simulink model "a"  (R2018b)
settings: Solver=VariableStepAuto  StartTime=0.0  StopTime=30  RelTol=1e-6
values from neighbouring files (symbols this model uses):
  H0 = 1000    [init.m]
  m = 100    [init.m]
  V0 = 250    [init.m]
undefined symbols (not defined in the file or in its folder): alfa, G, p, Wx, Wz, x0, Y, z0
libraries: simulink x1
settings Model: Creator=cool  LastModifiedBy=cool

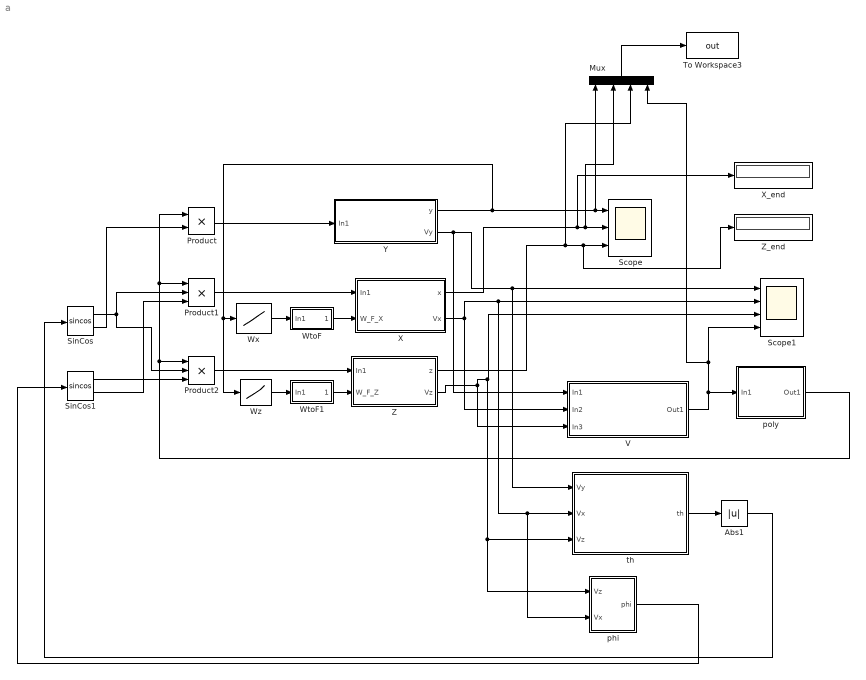
== system a ==
  Abs1 : Abs
  Mux : Mux
  Product : Product
  Product1 : Product  Inputs=3
  Product2 : Product  Inputs=3
  Scope : Scope  NumInputPorts=3
  Scope1 : Scope  NumInputPorts=4
  SinCos : Trigonometry  Operator=sincos
  SinCos1 : Trigonometry  Operator=sincos
  To Workspace3 : ToWorkspace  VariableName=out  SaveFormat=Timeseries  SampleTime=-1
  V : Subsystem
  WtoF : Subsystem
  WtoF1 : Subsystem
  Wx : Lookup_n-D  NumberOfTableDimensions=1  BreakpointsForDimension1=Y  Table=Wx  InterpMethod=Cubic spline  InternalRulePriority=Speed  RndMeth=Simplest  InputSameDT=on
  Wz : Lookup_n-D  NumberOfTableDimensions=1  BreakpointsForDimension1=Y  Table=Wz  InterpMethod=Cubic spline  InternalRulePriority=Speed  RndMeth=Simplest  InputSameDT=on
  X : Subsystem
  X_end : Display
  Y : Subsystem
  Z : Subsystem
  Z_end : Display
  "phi " : Subsystem
  "poly " : Subsystem
  th : Subsystem
  wires:
  Y/1(y) -> Wx/1, Wz/1, Scope/1, Mux/1
  X/1(x) -> Mux/2, Scope/2, X_end/1
  Z/1(z) -> Mux/3, Z_end/1, Scope/3
  Y/2(Vy) -> V/1(In1), th/1(Vy), Scope1/1
  X/2(Vx) -> "phi "/2(Vx), th/2(Vx), Scope1/2, V/2(In2)
  Z/2(Vz) -> "phi "/1(Vz), th/3(Vz), Scope1/3, V/3(In3)
  V/1(Out1) -> "poly "/1(In1), Mux/4, Scope1/4
  "poly "/1(Out1) -> Product2/1, Product/1, Product1/1
  th/1(th) -> Abs1/1
  SinCos/2 -> Product/2
  SinCos/1 -> Product1/2, Product2/2
  Product/1 -> Y/1(In1)
  Product2/1 -> Z/1(In1)
  Product1/1 -> X/1(In1)
  "phi "/1(phi) -> SinCos1/1
  Abs1/1 -> SinCos/1
  SinCos1/2 -> Product1/3
  SinCos1/1 -> Product2/3
  Mux/1 -> To Workspace3/1
  Wx/1 -> WtoF/1(In1)
  WtoF/1(Out1) -> X/2(W_F_X)
  Wz/1 -> WtoF1/1(In1)
  WtoF1/1(Out1) -> Z/2(W_F_Z)

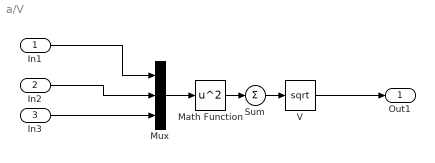
== system a/V ==
  In1 : Inport
  In2 : Inport  Port=2
  In3 : Inport  Port=3
  Math Function : Math  Operator=square  SaturateOnIntegerOverflow=on
  Mux : Mux  Inputs=3
  Sum : Sum  Inputs=+
  V : Sqrt  SaturateOnIntegerOverflow=on
  Out1 : Outport
  wires:
  Mux/1 -> Math Function/1
  In3/1 -> Mux/3
  Math Function/1 -> Sum/1
  In2/1 -> Mux/2
  Sum/1 -> V/1
  In1/1 -> Mux/1
  V/1 -> Out1/1

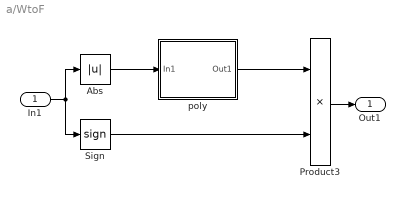
== system a/WtoF ==
  In1 : Inport
  Abs : Abs
  Product3 : Product
  Sign : Signum
  "poly " : Subsystem
  Out1 : Outport
  wires:
  In1/1 -> Sign/1, Abs/1
  Product3/1 -> Out1/1
  Sign/1 -> Product3/2
  Abs/1 -> "poly "/1(In1)
  "poly "/1(Out1) -> Product3/1

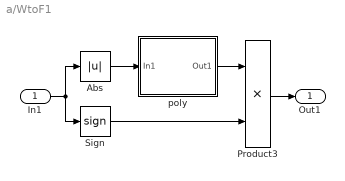
== system a/WtoF1 ==
  In1 : Inport
  Abs : Abs
  Product3 : Product
  Sign : Signum
  "poly " : Subsystem
  Out1 : Outport
  wires:
  Sign/1 -> Product3/2
  Product3/1 -> Out1/1
  In1/1 -> Abs/1, Sign/1
  "poly "/1(Out1) -> Product3/1
  Abs/1 -> "poly "/1(In1)

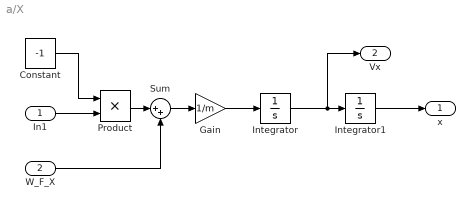
== system a/X ==
  In1 : Inport
  W_F_X : Inport  Port=2
  Constant : Constant  Value=-1
  Gain : Gain  Gain=1/m
  Integrator : Integrator  InitialCondition=V0*cos(alfa)
  Integrator1 : Integrator  InitialCondition=x0
  Product : Product
  Sum : Sum  Inputs=|++
  x : Outport
  Vx : Outport  Port=2
  wires:
  Integrator1/1 -> x/1
  Gain/1 -> Integrator/1
  In1/1 -> Product/2
  Constant/1 -> Product/1
  Integrator/1 -> Vx/1, Integrator1/1
  Product/1 -> Sum/1
  Sum/1 -> Gain/1
  W_F_X/1 -> Sum/2

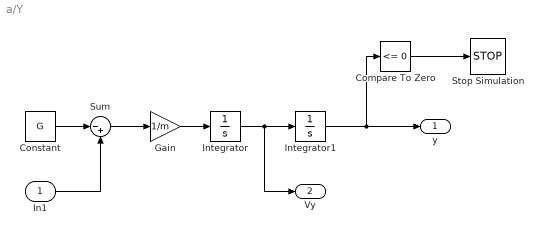
== system a/Y ==
  In1 : Inport
  Compare To Zero : simulink/Logic and Bit Operations/Compare To Zero  relop=<=  OutDataTypeStr=boolean
  Constant : Constant  Value=G
  Gain : Gain  Gain=1/m
  Integrator : Integrator
  Integrator1 : Integrator  InitialCondition=H0
  Stop Simulation : Stop
  Sum : Sum  Inputs=|-+
  y : Outport
  Vy : Outport  Port=2
  wires:
  Gain/1 -> Integrator/1
  Compare To Zero/1 -> Stop Simulation/1
  Integrator1/1 -> Compare To Zero/1, y/1
  Sum/1 -> Gain/1
  Constant/1 -> Sum/1
  In1/1 -> Sum/2
  Integrator/1 -> Vy/1, Integrator1/1

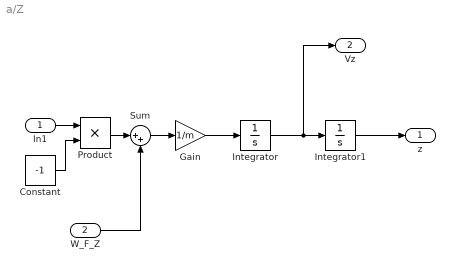
== system a/Z ==
  In1 : Inport
  W_F_Z : Inport  Port=2
  Constant : Constant  Value=-1
  Gain : Gain  Gain=1/m
  Integrator : Integrator  InitialCondition=V0*sin(alfa)
  Integrator1 : Integrator  InitialCondition=z0
  Product : Product
  Sum : Sum  Inputs=|++
  z : Outport
  Vz : Outport  Port=2
  wires:
  Gain/1 -> Integrator/1
  Integrator1/1 -> z/1
  In1/1 -> Product/1
  Constant/1 -> Product/2
  Integrator/1 -> Vz/1, Integrator1/1
  Product/1 -> Sum/1
  Sum/1 -> Gain/1
  W_F_Z/1 -> Sum/2

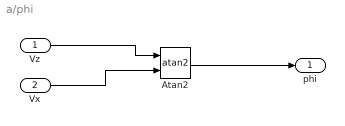
== system a/phi  ==
  Vz : Inport
  Vx : Inport  Port=2
  Atan2 : Trigonometry  Operator=atan2
  phi : Outport
  wires:
  Atan2/1 -> phi/1
  Vx/1 -> Atan2/2
  Vz/1 -> Atan2/1

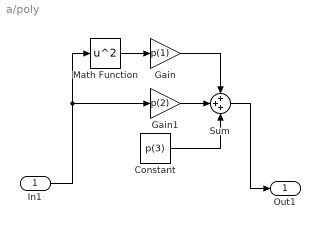
== system a/poly  ==
  In1 : Inport
  Constant : Constant  Value=p(3)
  Gain : Gain  Gain=p(1)
  Gain1 : Gain  Gain=p(2)
  Math Function : Math  Operator=square  SaturateOnIntegerOverflow=on
  Sum : Sum  Inputs=3
  Out1 : Outport
  wires:
  In1/1 -> Gain1/1, Math Function/1
  Constant/1 -> Sum/3
  Gain1/1 -> Sum/2
  Math Function/1 -> Gain/1
  Gain/1 -> Sum/1
  Sum/1 -> Out1/1

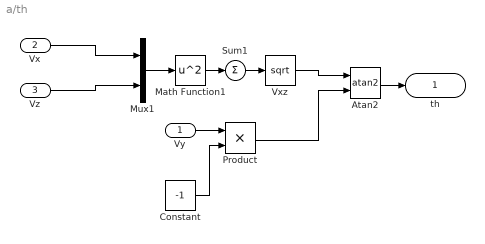
== system a/th ==
  Vy : Inport
  Vx : Inport  Port=2
  Vz : Inport  Port=3
  Atan2 : Trigonometry  Operator=atan2
  Constant : Constant  Value=-1
  Math Function1 : Math  Operator=square  SaturateOnIntegerOverflow=on
  Mux1 : Mux  Inputs=2
  Product : Product
  Sum1 : Sum  Inputs=+
  Vxz : Sqrt  SaturateOnIntegerOverflow=on
  th : Outport
  wires:
  Math Function1/1 -> Sum1/1
  Vx/1 -> Mux1/1
  Sum1/1 -> Vxz/1
  Vz/1 -> Mux1/2
  Mux1/1 -> Math Function1/1
  Vy/1 -> Product/1
  Constant/1 -> Product/2
  Atan2/1 -> th/1
  Vxz/1 -> Atan2/1
  Product/1 -> Atan2/2

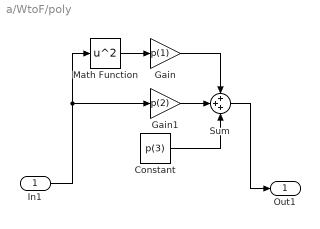
== system a/WtoF/poly  ==
  In1 : Inport
  Constant : Constant  Value=p(3)
  Gain : Gain  Gain=p(1)
  Gain1 : Gain  Gain=p(2)
  Math Function : Math  Operator=square  SaturateOnIntegerOverflow=on
  Sum : Sum  Inputs=3
  Out1 : Outport
  wires:
  In1/1 -> Gain1/1, Math Function/1
  Constant/1 -> Sum/3
  Gain1/1 -> Sum/2
  Math Function/1 -> Gain/1
  Gain/1 -> Sum/1
  Sum/1 -> Out1/1

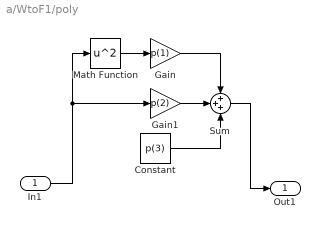
== system a/WtoF1/poly  ==
  In1 : Inport
  Constant : Constant  Value=p(3)
  Gain : Gain  Gain=p(1)
  Gain1 : Gain  Gain=p(2)
  Math Function : Math  Operator=square  SaturateOnIntegerOverflow=on
  Sum : Sum  Inputs=3
  Out1 : Outport
  wires:
  In1/1 -> Gain1/1, Math Function/1
  Constant/1 -> Sum/3
  Gain1/1 -> Sum/2
  Math Function/1 -> Gain/1
  Gain/1 -> Sum/1
  Sum/1 -> Out1/1
